simulink model "simula_processo_sem_integrador_1"  (R2017b)
settings: Solver=VariableStepAuto  StartTime=0.0  StopTime=5  RelTol=1e-3
settings Model: Creator=fernandopassold  LastModifiedBy=fernandopassold
settings CodeAppCC: StateflowObjectComments=on

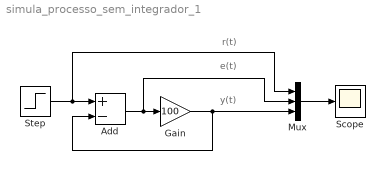
== system simula_processo_sem_integrador_1 ==
  note: y(t)
  note: e(t)
  note: r(t)
  Add : Sum  Inputs=+-
  Gain : Gain  Gain=100
  Mux : Mux  Inputs=3
  Scope : Scope
  Step : Step  SampleTime=0
  wires:
  Gain/1 -> Mux/3, Add/2
  Mux/1 -> Scope/1
  Add/1 -> Mux/2, Gain/1
  Step/1 -> Mux/1, Add/1
